simulink model "untitled"  (Simulink 6.5)
settings: Solver=ode45  StartTime=0.0  StopTime=80000  RelTol=1e-3
settings Model: Creator=ms44721  LastModifiedBy=ms44721

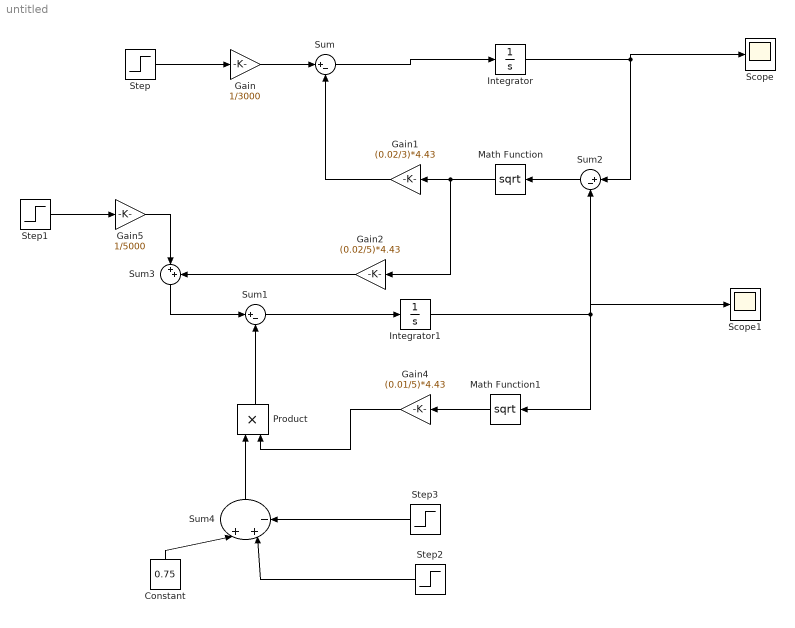
== system untitled ==
  Constant : Constant  Orientation=up  Value=0.75  OutDataType=sfix(16)  ConRadixGroup=Use specified scaling  OutScaling=2^0  SampleTime=inf  FramePeriod=inf
  Gain : Gain  Gain=1/3000
  Gain1 : Gain  Orientation=left  Gain=(0.02/3)*4.43
  Gain2 : Gain  Orientation=left  Gain=(0.02/5)*4.43
  Gain4 : Gain  Orientation=left  Gain=(0.01/5)*4.43
  Gain5 : Gain  Gain=1/5000
  Integrator : Integrator  LimitOutput=on  UpperSaturationLimit=10  LowerSaturationLimit=0
  Integrator1 : Integrator  LimitOutput=on  UpperSaturationLimit=10  LowerSaturationLimit=0
  Math Function : Math  Orientation=left  Operator=sqrt  SaturateOnIntegerOverflow=on
  Math Function1 : Math  Orientation=left  Operator=sqrt  SaturateOnIntegerOverflow=on
  Product : Product  Orientation=up  RndMeth=Zero
  Scope : Scope
  Scope1 : Scope
  Step : Step  After=30  SampleTime=0
  Step1 : Step  After=10  SampleTime=0
  Step2 : Step  Orientation=left  Time=20000  After=0.15  SampleTime=0
  Step3 : Step  Orientation=left  Time=40000  After=0.3  SampleTime=0
  Sum : Sum  Inputs=|+-
  Sum1 : Sum  Inputs=|+-
  Sum2 : Sum  Orientation=left  Inputs=|+-
  Sum3 : Sum  Orientation=down  Inputs=|++
  Sum4 : Sum  Orientation=up  Inputs=|++-
  wires:
  Step/1 -> Gain/1
  Sum/1 -> Integrator/1
  Integrator/1 -> Sum2/1, Scope/1
  Sum2/1 -> Math Function/1
  Math Function/1 -> Gain1/1, Gain2/1
  Sum1/1 -> Integrator1/1
  Integrator1/1 -> Sum2/2, Math Function1/1, Scope1/1
  Math Function1/1 -> Gain4/1
  Gain1/1 -> Sum/2
  Gain/1 -> Sum/1
  Gain2/1 -> Sum3/2
  Gain5/1 -> Sum3/1
  Step1/1 -> Gain5/1
  Sum3/1 -> Sum1/1
  Gain4/1 -> Product/2
  Product/1 -> Sum1/2
  Sum4/1 -> Product/1
  Constant/1 -> Sum4/1
  Step2/1 -> Sum4/2
  Step3/1 -> Sum4/3
